simulink model "templateVFreplay"  (R2019b)
settings: Solver=ode23tb  StartTime=0  StopTime=dataSim(l).Time(end)  FixedStep=Ts
model workspace (MAT data in the model file):
  AC8B_test_sdosession : sldodialogs.data.SessionData (value not decoded)
  tp34291882_bceb_4da8_b486_81ba615ab517 = [0 0.0333333 0.0666667 0.1 0.1333334 0.1666667 0.2 0.2333333 0.2666666 0.2999999 0.3333332 0.3666665 ... (13500 elements, 2700x5)]
  tp5fd81924_c6b2_4820_a4c1_c746ac51258e : object (value not decoded)
  tp61e2f470_2812_498a_af75_e87b8b944307 = [0 0.0333333 0.0666667 0.1 0.1333334 0.1666667 0.2 0.2333333 0.2666666 0.2999999 0.3333332 0.3666665 ... (13500 elements, 2700x5)]
  tpfa3056f0_c430_45b3_969f_b76cef1498ad : object (value not decoded)
undefined symbols (not defined in the file): dataSim, dyn, Fnom, g, gcbh, genTpd0, genTppd0, genTppq0, genTpq0, genXd, genXl, genXpd, genXppd, genXppq, genXpq, genXq, govDisable, ifd, init, j, l, MBase, p, sps_rtmsupport, sys, Tb1, Tc1, Vnom, vt
libraries: powerlib x28, modelLibrary x22, simulink x15, powerlib_meascontrol x5, spsST2AModel x4, GenLib x2, ideal_source x1
(part 4 of 4)

== system templateVFreplay/VF Replay/AVR/ST4B/ST4B Excitation System (Continuous)/Fex ==
  note: In<=0.433        Case 3
      | 0.433<In<0.75 Case 2
      | 0.75<=In<=1.0 Case 1
      | In>1.0               default
  In : Inport
  0.433<In<0.75 : Subsystem  TreatAsAtomicUnit=on
  0.75<=In<=1.0 : Subsystem  TreatAsAtomicUnit=on
  In<=0.433 : Subsystem  TreatAsAtomicUnit=on
  In>1.0 : Subsystem  TreatAsAtomicUnit=on
  Merge : Merge  Inputs=4
  Relational Operator : RelationalOperator  Operator=<=  RndMeth=Nearest  InputSameDT=on
  Relational Operator1 : RelationalOperator  Operator=<  RndMeth=Nearest  InputSameDT=on
  Relational Operator2 : RelationalOperator  Operator=<=  RndMeth=Nearest  InputSameDT=on
  Sum : Sum  Inputs=+++  AccumDataTypeStr=double  OutDataTypeStr=double  SaturateOnIntegerOverflow=on  InputSameDT=on
  Switch Case : SwitchCase  CaseConditions={1 2 3}
  input : Constant  Value=0.433
  input1 : Constant  Value=0.75
  input2 : Constant  Value=1.0
  Fex : Outport  VectorParamsAs1DForOutWhenUnconnected=off
  wires:
  Merge/1 -> Fex/1
  In/1 -> Relational Operator2/1, 0.75<=In<=1.0/1(In), 0.433<In<0.75/1(In), In<=0.433/1(In), Relational Operator1/1, Relational Operator/1  "In"
  0.75<=In<=1.0/1(f(In)) -> Merge/1
  0.433<In<0.75/1(f(In)) -> Merge/2
  In>1.0/1(f(In)) -> Merge/4
  In<=0.433/1(f(In)) -> Merge/3
  input1/1 -> Relational Operator1/2
  input2/1 -> Relational Operator2/2
  Relational Operator1/1 -> Sum/2
  Relational Operator/1 -> Sum/1
  Relational Operator2/1 -> Sum/3
  Sum/1 -> Switch Case/1
  Switch Case/1 -> 0.75<=In<=1.0/Action
  Switch Case/2 -> 0.433<In<0.75/Action
  Switch Case/3 -> In<=0.433/Action
  Switch Case/4 -> In>1.0/Action
  input/1 -> Relational Operator/2

== system templateVFreplay/VF Replay/AVR/ST4B/ST4B Excitation System (Continuous)/Fex1 ==
  Ve : Inport
  Ifd : Inport  Port=2
  Fcn : Fcn  Expr=u+(u==0)*eps
  Gain : Gain  Gain=Kc  SaturateOnIntegerOverflow=on  OutDataTypeStr=Inherit: Same as input  ParamDataTypeStr=Inherit: Same as input
  Product : Product  Inputs=*/  SaturateOnIntegerOverflow=on  RndMeth=Zero  InputSameDT=on  OutDataTypeStr=Inherit: Same as first input
  IN : Outport  VectorParamsAs1DForOutWhenUnconnected=off
  wires:
  Product/1 -> Gain/1
  Ifd/1 -> Product/1
  Fcn/1 -> Product/2
  Ve/1 -> Fcn/1
  Gain/1 -> IN/1  "In"

== system templateVFreplay/VF Replay/AVR/ST4B/ST4B Excitation System (Continuous)/S1 ==
  In1 : Inport
  Gain2 : Gain  Gain=Kpr
  Gain3 : Gain  Gain=Kir
  Integrator (Anti-windup) : Subsystem
      mask Display: dpoly([1],[1 0],'s')
  Saturation1 : Saturate  UpperLimit=Vrmax  LowerLimit=Vrmin
  Sum2 : Sum  Inputs=|++
  Out1 : Outport  VectorParamsAs1DForOutWhenUnconnected=off
  wires:
  Gain3/1 -> Integrator (Anti-windup)/1(u)
  In1/1 -> Gain3/1, Gain2/1
  Integrator (Anti-windup)/1(Out2) -> Sum2/2
  Gain2/1 -> Sum2/1
  Sum2/1 -> Integrator (Anti-windup)/2(ctrlOutput1), Saturation1/1
  Saturation1/1 -> Out1/1

== system templateVFreplay/VF Replay/AVR/ST4B/ST4B Excitation System (Continuous)/Subsystem2 ==
  note: Kp*Vt
  Vt : Inport
  Vt_Ang : Inport  Port=2
  It : Inport  Port=3
  It_Ang : Inport  Port=4
  Complex to Magnitude : ComplexToMagnitudeAngle  Output=Magnitude
  Current Source Gain : Constant  Value=Ki
  Gain : Gain  Gain=j
  Leakage Reactance : Constant  Value=Xl
  Magnitude-Angle to Complex : MagnitudeAngleToComplex
  Magnitude-Angle to Complex1 : MagnitudeAngleToComplex
  Magnitude-Angle to Complex2 : MagnitudeAngleToComplex
  Potential Source Gain : Constant  Value=Kp
  Potential Source Phase Angle : Constant  Value=Angp
  Product1 : Product  SaturateOnIntegerOverflow=on  RndMeth=Zero  InputSameDT=on  OutDataTypeStr=Inherit: Same as first input
  Product2 : Product  SaturateOnIntegerOverflow=on  RndMeth=Zero  InputSameDT=on  OutDataTypeStr=Inherit: Same as first input
  Product3 : Product  SaturateOnIntegerOverflow=on  RndMeth=Zero  InputSameDT=on  OutDataTypeStr=Inherit: Same as first input
  Sum5 : Sum  Inputs=|++
  Sum6 : Sum  Inputs=++|
  Ve : Outport  VectorParamsAs1DForOutWhenUnconnected=off
  wires:
  Magnitude-Angle to Complex2/1 -> Product2/1
  Potential Source Phase Angle/1 -> Magnitude-Angle to Complex/2
  Magnitude-Angle to Complex1/1 -> Product1/2
  Potential Source Gain/1 -> Magnitude-Angle to Complex/1
  Product1/1 -> Sum5/1
  Product2/1 -> Sum5/2
  Sum5/1 -> Complex to Magnitude/1
  Vt/1 -> Magnitude-Angle to Complex1/1
  Complex to Magnitude/1 -> Ve/1  "Ve"
  Magnitude-Angle to Complex/1 -> Product3/1, Product1/1
  Leakage Reactance/1 -> Product3/2
  Product3/1 -> Sum6/2  "Kp*XL"
  Current Source Gain/1 -> Sum6/1
  Sum6/1 -> Gain/1  "Ki+Kp*XL"
  Gain/1 -> Product2/2
  It/1 -> Magnitude-Angle to Complex2/1
  Vt_Ang/1 -> Magnitude-Angle to Complex1/2
  It_Ang/1 -> Magnitude-Angle to Complex2/2

== system templateVFreplay/VF Replay/AVR/ST4B/ST4B Excitation System (Continuous)/Subsystem4 ==
  In1 : Inport
  Gain2 : Gain  Gain=Kpm
  Gain3 : Gain  Gain=Kim
  Integrator (Anti-windup) : Subsystem
      mask Display: dpoly([1],[1 0],'s')
  Saturation1 : Saturate  UpperLimit=Vmmax  LowerLimit=Vmmin
  Sum2 : Sum  Inputs=|++
  Out1 : Outport  VectorParamsAs1DForOutWhenUnconnected=off
  wires:
  Gain3/1 -> Integrator (Anti-windup)/1(u)
  Saturation1/1 -> Out1/1
  Gain2/1 -> Sum2/1
  Integrator (Anti-windup)/1(Out2) -> Sum2/2
  In1/1 -> Gain2/1, Gain3/1
  Sum2/1 -> Integrator (Anti-windup)/2(ctrlOutput1), Saturation1/1

== system templateVFreplay/VF Replay/AVR/ST4B/ST4B Excitation System (Continuous)/k//(tau.s+1)1 ==
  u : Inport
  1/(taus+1) : Subsystem  mask{tau=tau, vmax=vmax, vmin=vmin}
      mask prompts: tau "Time Constant"
      mask init:
      | h = gcbh;
      | 
      | qq = get(h,'MaskValues');
      | 
      | if eval(qq{1}) == 0
      |     
      |     set(h,'Commented','through');
      |     
      | else
      |     
      |     set(h,'Commented','off');
      |     
      | end
  k : Gain  Gain=k
  y : Outport  VectorParamsAs1DForOutWhenUnconnected=off
  wires:
  1/(taus+1)/1(y) -> y/1
  u/1 -> k/1
  k/1 -> 1/(taus+1)/1(u)

== system templateVFreplay/VF Replay/GENERATION/GENROU_TERMINAL/freqMeas/S0 ==
  u : Inport
  Gain : Gain  Gain=1/1e-2
  Gain1 : Gain  Gain=1e-2
  Integrator : Integrator
  Sum : Sum  Inputs=|+-
  y : Outport  InitialOutput=0  VectorParamsAs1DForOutWhenUnconnected=off
  wires:
  Gain1/1 -> y/1
  Integrator/1 -> Sum/2
  Gain/1 -> Integrator/1, Gain1/1
  Sum/1 -> Gain/1
  u/1 -> Sum/1

== system templateVFreplay/VF Replay/GENERATION/GENROU_TERMINAL/freqMeas/S1 ==
  u : Inport
  Gain2 : Gain  Gain=100
  Integrator1 : Integrator
  Sum : Sum  Inputs=|+-
  y : Outport  InitialOutput=0  VectorParamsAs1DForOutWhenUnconnected=off
  wires:
  u/1 -> Sum/1
  Sum/1 -> Gain2/1
  Integrator1/1 -> y/1, Sum/2
  Gain2/1 -> Integrator1/1

== system templateVFreplay/VF Replay/GENERATION/GENROU_TRANSFORMER/freqMeas/S0 ==
  u : Inport
  Gain : Gain  Gain=1/1e-2
  Gain1 : Gain  Gain=1e-2
  Integrator : Integrator
  Sum : Sum  Inputs=|+-
  y : Outport  InitialOutput=0  VectorParamsAs1DForOutWhenUnconnected=off
  wires:
  u/1 -> Sum/1
  Sum/1 -> Gain/1
  Gain/1 -> Gain1/1, Integrator/1
  Integrator/1 -> Sum/2
  Gain1/1 -> y/1

== system templateVFreplay/VF Replay/GENERATION/GENROU_TRANSFORMER/freqMeas/S1 ==
  u : Inport
  Gain2 : Gain  Gain=100
  Integrator1 : Integrator
  Sum : Sum  Inputs=|+-
  y : Outport  InitialOutput=0  VectorParamsAs1DForOutWhenUnconnected=off
  wires:
  Gain2/1 -> Integrator1/1
  Integrator1/1 -> Sum/2, y/1
  Sum/1 -> Gain2/1
  u/1 -> Sum/1

== system templateVFreplay/VF Replay/GENERATION/GENSAL_TRANSFORMER/freqMeas/S0 ==
  u : Inport
  Gain : Gain  Gain=1/1e-2
  Gain1 : Gain  Gain=1e-2
  Integrator : Integrator
  Sum : Sum  Inputs=|+-
  y : Outport  InitialOutput=0  VectorParamsAs1DForOutWhenUnconnected=off
  wires:
  Gain1/1 -> y/1
  Integrator/1 -> Sum/2
  Gain/1 -> Integrator/1, Gain1/1
  Sum/1 -> Gain/1
  u/1 -> Sum/1

== system templateVFreplay/VF Replay/GENERATION/GENSAL_TRANSFORMER/freqMeas/S1 ==
  u : Inport
  Gain2 : Gain  Gain=100
  Integrator1 : Integrator
  Sum : Sum  Inputs=|+-
  y : Outport  InitialOutput=0  VectorParamsAs1DForOutWhenUnconnected=off
  wires:
  u/1 -> Sum/1
  Sum/1 -> Gain2/1
  Integrator1/1 -> y/1, Sum/2
  Gain2/1 -> Integrator1/1

== system templateVFreplay/VF Replay/GENERATION/GENTPJ_TERMINAL/freqMeas/S0 ==
  u : Inport
  Gain : Gain  Gain=1/1e-2
  Gain1 : Gain  Gain=1e-2
  Integrator : Integrator
  Sum : Sum  Inputs=|+-
  y : Outport  InitialOutput=0  VectorParamsAs1DForOutWhenUnconnected=off
  wires:
  Gain1/1 -> y/1
  Integrator/1 -> Sum/2
  Gain/1 -> Integrator/1, Gain1/1
  Sum/1 -> Gain/1
  u/1 -> Sum/1

== system templateVFreplay/VF Replay/GENERATION/GENTPJ_TERMINAL/freqMeas/S1 ==
  u : Inport
  Gain2 : Gain  Gain=100
  Integrator1 : Integrator
  Sum : Sum  Inputs=|+-
  y : Outport  InitialOutput=0  VectorParamsAs1DForOutWhenUnconnected=off
  wires:
  u/1 -> Sum/1
  Sum/1 -> Gain2/1
  Integrator1/1 -> y/1, Sum/2
  Gain2/1 -> Integrator1/1

== system templateVFreplay/VF Replay/GENERATION/GENTPJ_TRANSFORMER/freqMeas/S0 ==
  u : Inport
  Gain : Gain  Gain=1/1e-2
  Gain1 : Gain  Gain=1e-2
  Integrator : Integrator
  Sum : Sum  Inputs=|+-
  y : Outport  InitialOutput=0  VectorParamsAs1DForOutWhenUnconnected=off
  wires:
  u/1 -> Sum/1
  Sum/1 -> Gain/1
  Gain/1 -> Gain1/1, Integrator/1
  Integrator/1 -> Sum/2
  Gain1/1 -> y/1

== system templateVFreplay/VF Replay/GENERATION/GENTPJ_TRANSFORMER/freqMeas/S1 ==
  u : Inport
  Gain2 : Gain  Gain=100
  Integrator1 : Integrator
  Sum : Sum  Inputs=|+-
  y : Outport  InitialOutput=0  VectorParamsAs1DForOutWhenUnconnected=off
  wires:
  Gain2/1 -> Integrator1/1
  Integrator1/1 -> Sum/2, y/1
  Sum/1 -> Gain2/1
  u/1 -> Sum/1

== system templateVFreplay/VF Replay/GOV/GGOV1/General Governor (Continuous) /Engine Power vs Speed ==
  u : Inport
  Droop3 : Gain  Gain=Dm
  Pmwset6 : Constant  Value=Dm
  Pmwset7 : Constant  Value=0
  Switch : Switch  Criteria=u2 > Threshold  ZeroCross=off
  y : Outport  VectorParamsAs1DForOutWhenUnconnected=off
  wires:
  u/1 -> Switch/1
  Droop3/1 -> y/1
  Switch/1 -> Droop3/1
  Pmwset7/1 -> Switch/3
  Pmwset6/1 -> Switch/2

== system templateVFreplay/VF Replay/GOV/GGOV1/General Governor (Continuous) /Fuel Flow Factor ==
  u : Inport
  Math Function : Math  Operator=pow  SaturateOnIntegerOverflow=on
  Pmwset6 : Constant  Value=Dm
  Pmwset7 : Constant  Value=0
  Pmwset8 : Constant  Value=Dm
  Switch : Switch  Criteria=u2 > Threshold  ZeroCross=off
  y : Outport  VectorParamsAs1DForOutWhenUnconnected=off
  wires:
  Pmwset7/1 -> Switch/1
  u/1 -> Switch/3
  Math Function/1 -> y/1
  Pmwset8/1 -> Math Function/2
  Switch/1 -> Math Function/1
  Pmwset6/1 -> Switch/2

== system templateVFreplay/VF Replay/GOV/GGOV1/General Governor (Continuous) /S0 ==
  In : Inport
  1/Tpelec : Gain  Gain=1/Tpelec
  Integrator : Integrator
  Sum : Sum  Inputs=|+-
  Out : Outport  InitialOutput=0  VectorParamsAs1DForOutWhenUnconnected=off
  wires:
  Sum/1 -> 1/Tpelec/1
  1/Tpelec/1 -> Integrator/1
  In/1 -> Sum/1
  Integrator/1 -> Sum/2, Out/1

== system templateVFreplay/VF Replay/GOV/GGOV1/General Governor (Continuous) /S1 ==
  u : Inport
  Droop1 : Gain  Gain=Kpgov
  S1_TF : Subsystem
      mask Display: disp('s K_{dgov} / (1 + s T_{dgov})','texmode','on');
  Sum4 : Sum  Inputs=++|
  y : Outport  InitialOutput=0  VectorParamsAs1DForOutWhenUnconnected=off
  wires:
  Sum4/1 -> y/1  "Pm0*Kpgov"
  S1_TF/1(y) -> Sum4/1  "0"
  Droop1/1 -> Sum4/2
  u/1 -> Droop1/1, S1_TF/1(u)

== system templateVFreplay/VF Replay/GOV/GGOV1/General Governor (Continuous) /S2 ==
  u : Inport
  Droop2 : Gain  Gain=Kigov/Kpgov
  Integrator : Integrator
  y : Outport  InitialOutput=0  VectorParamsAs1DForOutWhenUnconnected=off
  wires:
  Integrator/1 -> y/1
  Droop2/1 -> Integrator/1
  u/1 -> Droop2/1

== system templateVFreplay/VF Replay/GOV/GGOV1/General Governor (Continuous) /S3 ==
  u : Inport
  Droop2 : Gain  Gain=1/Tact
  Integrator : Integrator  InitialCondition=1
  Saturation3 : Saturate  Commented=through  UpperLimit=ropen  LowerLimit=rclose
      settings: AttributesFormatString=|
      | %<UpperLimit>
      | %<LowerLimit>
  y : Outport  InitialOutput=0  VectorParamsAs1DForOutWhenUnconnected=off
  wires:
  u/1 -> Droop2/1
  Droop2/1 -> Saturation3/1
  Saturation3/1 -> Integrator/1
  Integrator/1 -> y/1

== system templateVFreplay/VF Replay/GOV/GGOV1/General Governor (Continuous) /S4 ==
  u : Inport
  Gain : Gain  Gain=1/Tb
  Gain1 : Gain  Gain=Tc
  Integrator : Integrator  InitialCondition=1
  Sum : Sum  Inputs=|+-
  Sum1 : Sum  Inputs=++|
  y : Outport  InitialOutput=0  VectorParamsAs1DForOutWhenUnconnected=off
  wires:
  Sum1/1 -> y/1
  Gain/1 -> Integrator/1, Gain1/1
  Sum/1 -> Gain/1
  u/1 -> Sum/1  "Pm0"
  Integrator/1 -> Sum1/2, Sum/2
  Gain1/1 -> Sum1/1

== system templateVFreplay/VF Replay/GOV/GGOV1/General Governor (Continuous) /S5 ==
  u : Inport
  1/Tfload : Gain  Gain=1/Tfload
  Integrator : Integrator
  Sum : Sum  Inputs=|+-
  y : Outport  InitialOutput=0  VectorParamsAs1DForOutWhenUnconnected=off
  wires:
  Sum/1 -> 1/Tfload/1
  1/Tfload/1 -> Integrator/1
  u/1 -> Sum/1
  Integrator/1 -> Sum/2, y/1

== system templateVFreplay/VF Replay/GOV/GGOV1/General Governor (Continuous) /S6 ==
  u : Inport
  Droop2 : Gain  Gain=Kiload/Kpload
  Integrator : Integrator
  y : Outport  InitialOutput=0  VectorParamsAs1DForOutWhenUnconnected=off
  wires:
  u/1 -> Droop2/1
  Droop2/1 -> Integrator/1
  Integrator/1 -> y/1

== system templateVFreplay/VF Replay/GOV/GGOV1/General Governor (Continuous) /S7 ==
  u : Inport
  Gain1 : Gain  Gain=Kimw
  Integrator : Integrator  UpperSaturationLimit=1.1*r  LowerSaturationLimit=-1.1*r
      settings: AttributesFormatString=|
      | %<UpperSaturationLimit>
      | %<LowerSaturationLimit>
  y : Outport  InitialOutput=0  VectorParamsAs1DForOutWhenUnconnected=off
  wires:
  u/1 -> Gain1/1
  Gain1/1 -> Integrator/1
  Integrator/1 -> y/1

== system templateVFreplay/VF Replay/GOV/GGOV1/General Governor (Continuous) /S8 ==
  u : Inport
  Gain : Gain  Gain=1/Ta
  Integrator : Integrator
  Sum : Sum  Inputs=|+-
  y : Outport  InitialOutput=0  VectorParamsAs1DForOutWhenUnconnected=off
  wires:
  Gain/1 -> Integrator/1, y/1
  u/1 -> Sum/1
  Sum/1 -> Gain/1
  Integrator/1 -> Sum/2

== system templateVFreplay/VF Replay/GOV/GGOV1/General Governor (Continuous) /S9 ==
  u : Inport
  Gain : Gain  Gain=1/Tsb
  Gain1 : Gain  Gain=Tsa
  Integrator : Integrator
  Sum : Sum  Inputs=|+-
  Sum1 : Sum  Inputs=++|
  y : Outport  InitialOutput=0  VectorParamsAs1DForOutWhenUnconnected=off
  wires:
  Gain1/1 -> Sum1/1
  Integrator/1 -> Sum/2, Sum1/2
  u/1 -> Sum/1  "Pm0/Kturb+wfnl"
  Sum/1 -> Gain/1
  Gain/1 -> Integrator/1, Gain1/1
  Sum1/1 -> y/1

== system templateVFreplay/VF Replay/GOV/GGOV1/General Governor (Continuous) /Subsystem ==
  Clock : Clock
  Memory : Memory  InitialCondition=-0.2
  Sum13 : Sum  Inputs=|+-
  dT : Outport  VectorParamsAs1DForOutWhenUnconnected=off
  wires:
  Sum13/1 -> dT/1
  Clock/1 -> Sum13/1, Memory/1
  Memory/1 -> Sum13/2

== system templateVFreplay/VF Replay/GOV/GGOV1/General Governor (Continuous) /Subsystem1 ==
  fsrt : Inport
  fsra : Inport  Port=2
  fsrn : Inport  Port=3
  Constant : Constant  Value=init*100
  Low Value Select : MinMax  Inputs=3  ZeroCross=off
  Sum : Sum  Inputs=|+-
  Sum1 : Sum  Inputs=|++
  Unit Delay : UnitDelay  SampleTime=-1  HasFrameUpgradeWarning=on
  Out1 : Outport  VectorParamsAs1DForOutWhenUnconnected=off
  wires:
  fsra/1 -> Low Value Select/2
  fsrt/1 -> Low Value Select/1
  Unit Delay/1 -> Out1/1
  fsrn/1 -> Sum/1
  Sum/1 -> Low Value Select/3
  Low Value Select/1 -> Sum1/1
  Sum1/1 -> Unit Delay/1
  Constant/1 -> Sum1/2, Sum/2

== system templateVFreplay/VF Replay/GOV/IEEEG3/Hydro Turbine//Governor (Continuous)/S0 ==
  u : Inport
  1/Tp : Gain  Gain=1/Tp
  Integrator : Integrator
  Sum : Sum  Inputs=|+-
  y : Outport  VectorParamsAs1DForOutWhenUnconnected=off
  wires:
  Integrator/1 -> y/1, Sum/2
  u/1 -> Sum/1
  1/Tp/1 -> Integrator/1
  Sum/1 -> 1/Tp/1

== system templateVFreplay/VF Replay/GOV/IEEEG3/Hydro Turbine//Governor (Continuous)/S2 ==
  u : Inport
  Gain : Gain  Gain=1/Tr
  Gain1 : Gain  Gain=Tr
  Gain2 : Gain  Gain=Rtemp
  Integrator : Integrator
  Sum : Sum  Inputs=|+-
  y : Outport  InitialOutput=0  VectorParamsAs1DForOutWhenUnconnected=off
  wires:
  Gain1/1 -> y/1
  Integrator/1 -> Sum/2
  Gain/1 -> Gain1/1, Integrator/1
  Sum/1 -> Gain/1
  u/1 -> Gain2/1
  Gain2/1 -> Sum/1

== system templateVFreplay/VF Replay/GOV/IEEEG3/Hydro Turbine//Governor (Continuous)/S3 ==
  u : Inport
  Gain : Gain  Gain=1/(Bturb*Tw)
  Gain1 : Gain  Gain=Aturb*Tw
  Gain2 : Gain  Gain=Kturb
  Integrator : Integrator  InitialCondition=1
  Sum : Sum  Inputs=|+-
  Sum1 : Sum  Inputs=++|
  y : Outport  InitialOutput=0  VectorParamsAs1DForOutWhenUnconnected=off
  wires:
  u/1 -> Gain2/1
  Sum1/1 -> y/1
  Gain/1 -> Gain1/1, Integrator/1
  Sum/1 -> Gain/1
  Gain2/1 -> Sum/1
  Integrator/1 -> Sum1/2, Sum/2
  Gain1/1 -> Sum1/1

== system templateVFreplay/VF Replay/PSS/PSS1A/Power System Stabilize 1A (Continuous)/(ta.s+1)//(tb.s+1)1 ==
  note: disable integrator and pass through signal if tb is zero
  u : Inport
  Constant : Constant  Value=tb
  Gain : Gain  Gain=1/(tb+eps)
  Gain1 : Gain  Gain=ta
  Integrator : Integrator
  Sum : Sum  Inputs=|+-
  Sum1 : Sum  Inputs=++|
  Switch : Switch  Criteria=u2 > Threshold
  Switch1 : Switch  Criteria=u2 > Threshold
  y : Outport  VectorParamsAs1DForOutWhenUnconnected=off
  wires:
  Switch1/1 -> y/1
  Sum1/1 -> Switch1/1
  Switch/1 -> Integrator/1
  Constant/1 -> Switch/2, Switch/3, Switch1/2
  u/1 -> Sum/1, Switch1/3
  Integrator/1 -> Sum/2, Sum1/2
  Gain1/1 -> Sum1/1
  Gain/1 -> Gain1/1, Switch/1
  Sum/1 -> Gain/1

== system templateVFreplay/VF Replay/PSS/PSS1A/Power System Stabilize 1A (Continuous)/S3_1 ==
  u : Inport
  1/A1 : Gain  Gain=1/A1
  Gain3 : Gain  Commented=on  Gain=A1/A2
  Gain4 : Gain  Commented=on  Gain=1/A2
  Gain5 : Gain  Commented=on  Gain=1/A2
  Integrator : Integrator
  Integrator2 : Integrator  Commented=on
  Integrator3 : Integrator  Commented=on
  Sum : Sum  Inputs=|+-
  Sum2 : Sum  Commented=on  Inputs=|+-
  Sum3 : Sum  Commented=on  Inputs=|++
  y : Outport  InitialOutput=0  VectorParamsAs1DForOutWhenUnconnected=off
  wires:
  Integrator/1 -> Sum/2, y/1
  u/1 -> Sum/1
  1/A1/1 -> Integrator/1
  Sum/1 -> 1/A1/1
  Gain4/1 -> Sum3/1
  Gain3/1 -> Sum3/2
  Sum3/1 -> Sum2/2  "Vs0/A2"
  Gain5/1 -> Sum2/1
  Sum2/1 -> Integrator2/1
  Integrator2/1 -> Gain3/1, Integrator3/1
  Integrator3/1 -> Gain4/1
  ? -> Gain5/1

== system templateVFreplay/VF Replay/PSS/PSS2A/Power System Stabilizer 2A (Continuous) /T9 ~= 0 ==
  u : Inport
  Filter1 : Subsystem
      mask Display: disp('(1 + s T_8) / (1 + s T_9)^m','texmode','on');
  y : Outport  VectorParamsAs1DForOutWhenUnconnected=off
  wires:
  u/1 -> Filter1/1(In1)
  Filter1/1(Out1) -> y/1

== system templateVFreplay/VF Replay/PSS/PSS2B/Power System Stabilizer 2B (Continuous) /T9 ~= 0 ==
  u : Inport
  Filter1 : Subsystem
      mask Display: disp('(1 + s T_8) / (1 + s T_9)^m','texmode','on');
  y : Outport  VectorParamsAs1DForOutWhenUnconnected=off
  wires:
  u/1 -> Filter1/1(In1)
  Filter1/1(Out1) -> y/1

== system templateVFreplay/VF Replay/AVR/REXS/Rotating Excitation System (Continuous) /S2 + S8/S2 ==
  In : Inport
  Tb1 = 0 : Subsystem  VariantControl=Tb1Zero
  Tb1 ~= 0 : Subsystem  VariantControl=Tb1NotZero
  Out : Outport  VectorParamsAs1DForOutWhenUnconnected=off

== system templateVFreplay/VF Replay/AVR/REXS/Rotating Excitation System (Continuous) /S2 + S8/S8 ==
  In : Inport
  Tb2 = 0 : Subsystem  VariantControl=Tb2Zero
  Tb2 ~= 0 : Subsystem  VariantControl=Tb2NotZero
  Out : Outport  VectorParamsAs1DForOutWhenUnconnected=off

== system templateVFreplay/VF Replay/AVR/ST1A/ST1A Excitation System/Model/(ta.s+1)//(tb.s+1)1 ==
  note: disable integrator and pass through signal if tb is zero
  u : Inport
  Constant : Constant  Value=tb
  Gain : Gain  Gain=1/(tb+eps)
  Gain1 : Gain  Gain=ta
  Integrator : Integrator
  Sum : Sum  Inputs=|+-
  Sum1 : Sum  Inputs=++|
  Switch : Switch  Criteria=u2 > Threshold
  Switch1 : Switch  Criteria=u2 > Threshold
  y : Outport  VectorParamsAs1DForOutWhenUnconnected=off
  wires:
  Switch1/1 -> y/1
  Sum1/1 -> Switch1/1
  Switch/1 -> Integrator/1
  Constant/1 -> Switch/2, Switch/3, Switch1/2
  u/1 -> Sum/1, Switch1/3
  Integrator/1 -> Sum/2, Sum1/2
  Gain1/1 -> Sum1/1
  Gain/1 -> Gain1/1, Switch/1
  Sum/1 -> Gain/1

== system templateVFreplay/VF Replay/AVR/ST1A/ST1A Excitation System/Model/Subsystem ==
  note: Vt.VRmin
  Efd : Inport
  Vt : Inport  Port=2
  Ifd : Inport  Port=3
  Gain2 : Gain  Gain=p.kc  SaturateOnIntegerOverflow=on  OutDataTypeStr=Inherit: Same as input  ParamDataTypeStr=Inherit: Same as input
  Gain5 : Gain  Gain=p.vrmax  SaturateOnIntegerOverflow=on  OutDataTypeStr=Inherit: Same as input  ParamDataTypeStr=Inherit: Same as input
  Gain6 : Gain  Gain=p.vrmin  SaturateOnIntegerOverflow=on  OutDataTypeStr=Inherit: Same as input  ParamDataTypeStr=Inherit: Same as input
  Saturation Dynamic : simulink/Discontinuities/Saturation Dynamic  OutMin=[]  OutMax=[]  OutDataTypeStr=Inherit: Same as second input  OutDataType=fixdt(1, 16)  OutScaling=2^-10  DoSatur=off
  Sum5 : Sum  Inputs=+-  SaturateOnIntegerOverflow=on  InputSameDT=on  OutDataTypeStr=Inherit: Same as first input
  Efd1 : Outport  VectorParamsAs1DForOutWhenUnconnected=off
  wires:
  Gain2/1 -> Sum5/2
  Ifd/1 -> Gain2/1  "Field current Ifd (pu)"
  Efd/1 -> Saturation Dynamic/2  "Field voltage Efd (pu)"
  Gain5/1 -> Sum5/1
  Vt/1 -> Gain6/1, Gain5/1  "Terminal voltage Vt (pu)"
  Saturation Dynamic/1 -> Efd1/1
  Sum5/1 -> Saturation Dynamic/1
  Gain6/1 -> Saturation Dynamic/3

== system templateVFreplay/VF Replay/AVR/ST1A/ST1A Excitation System/Model/const ==
  Constant : Constant  Value=0
  Integrator : Integrator
  y : Outport  VectorParamsAs1DForOutWhenUnconnected=off
  wires:
  Constant/1 -> Integrator/1
  Integrator/1 -> y/1

== system templateVFreplay/VF Replay/AVR/ST1A/ST1A Excitation System/Model/k.s//(tau.s+1) ==
  note: disable integrator and pass through signal if tau is zero
  u : Inport
  Constant : Constant  Value=tau
  Constant1 : Constant  Value=0
  Gain : Gain  Gain=1/(tau+eps)
  Gain1 : Gain  Gain=k
  Integrator : Integrator
  Sum : Sum  Inputs=|+-
  Switch : Switch  Criteria=u2 > Threshold
  Switch1 : Switch  Criteria=u2 > Threshold
  y : Outport  VectorParamsAs1DForOutWhenUnconnected=off
  wires:
  Gain1/1 -> Switch1/1
  Switch1/1 -> y/1
  Switch/1 -> Gain1/1, Integrator/1
  Gain/1 -> Switch/1
  Constant/1 -> Switch/2, Switch/3, Switch1/2
  Sum/1 -> Gain/1
  u/1 -> Sum/1
  Integrator/1 -> Sum/2
  Constant1/1 -> Switch1/3

== system templateVFreplay/VF Replay/AVR/ST1A/ST1A Excitation System/Model/k//(tau.s+1)1 ==
  u : Inport
  1/(taus+1) : Subsystem  mask{tau=tau, vmax=vmax, vmin=vmin}
      mask prompts: tau "Time Constant"
  k : Gain  Gain=k
  y : Outport  VectorParamsAs1DForOutWhenUnconnected=off
  wires:
  k/1 -> 1/(taus+1)/1(u)
  u/1 -> k/1
  1/(taus+1)/1(y) -> y/1

== system templateVFreplay/VF Replay/AVR/ST4B/ST4B Excitation System (Continuous)/Fex/0.433<In<0.75 ==
  In : Inport
  Action Port : ActionPort  InitializeStates=reset  ActionPortLabel=case [ 2 ]:
  Math Function : Math  Operator=square  SaturateOnIntegerOverflow=on
  Math Function1 : Math  Operator=sqrt  SaturateOnIntegerOverflow=on
  Sum : Sum  Inputs=+-|  SaturateOnIntegerOverflow=on  InputSameDT=on  OutDataTypeStr=Inherit: Same as first input
  input2 : Constant  Value=0.75
  f(In) : Outport  VectorParamsAs1DForOutWhenUnconnected=off
  wires:
  Math Function1/1 -> f(In)/1
  In/1 -> Math Function/1
  Math Function/1 -> Sum/2
  input2/1 -> Sum/1
  Sum/1 -> Math Function1/1

== system templateVFreplay/VF Replay/AVR/ST4B/ST4B Excitation System (Continuous)/Fex/0.75<=In<=1.0 ==
  In : Inport
  Action Port : ActionPort  InitializeStates=reset  ActionPortLabel=case [ 1 ]:
  Gain : Gain  Gain=1.732  SaturateOnIntegerOverflow=on  OutDataTypeStr=Inherit: Same as input  ParamDataTypeStr=Inherit: Same as input
  Sum : Sum  Inputs=+-|  SaturateOnIntegerOverflow=on  InputSameDT=on  OutDataTypeStr=Inherit: Same as first input
  input2 : Constant  Value=1.0
  f(In) : Outport  VectorParamsAs1DForOutWhenUnconnected=off
  wires:
  Gain/1 -> f(In)/1
  Sum/1 -> Gain/1
  input2/1 -> Sum/1
  In/1 -> Sum/2

== system templateVFreplay/VF Replay/AVR/ST4B/ST4B Excitation System (Continuous)/Fex/In<=0.433 ==
  In : Inport
  Action Port : ActionPort  InitializeStates=reset  ActionPortLabel=case [ 3 ]:
  Gain : Gain  Gain=0.577  SaturateOnIntegerOverflow=on  OutDataTypeStr=Inherit: Same as input  ParamDataTypeStr=Inherit: Same as input
  Sum : Sum  Inputs=+-|  SaturateOnIntegerOverflow=on  InputSameDT=on  OutDataTypeStr=Inherit: Same as first input
  input2 : Constant  Value=1.0
  f(In) : Outport  VectorParamsAs1DForOutWhenUnconnected=off
  wires:
  Sum/1 -> f(In)/1
  input2/1 -> Sum/1
  Gain/1 -> Sum/2
  In/1 -> Gain/1

== system templateVFreplay/VF Replay/AVR/ST4B/ST4B Excitation System (Continuous)/Fex/In>1.0 ==
  Action Port : ActionPort  InitializeStates=reset  ActionPortLabel=default:
  input2 : Constant  Value=0
  f(In) : Outport  InitialOutput=0  VectorParamsAs1DForOutWhenUnconnected=off
  wires:
  input2/1 -> f(In)/1

== system templateVFreplay/VF Replay/AVR/ST4B/ST4B Excitation System (Continuous)/S1/Integrator (Anti-windup) ==
  u : Inport
  ctrlOutput1 : Inport  Port=2
  Compare To Constant : simulink/Logic and Bit Operations/Compare To Constant  relop=>=  const=Vrmax  OutDataTypeStr=boolean
  Compare To Constant1 : simulink/Logic and Bit Operations/Compare To Constant  relop=<=  const=Vrmin  OutDataTypeStr=boolean
  Constant : Constant  Value=0
  Integrator : Integrator
  Logical Operator : Logic  Operator=OR  AllPortsSameDT=off  OutDataTypeStr=boolean
  Switch : Switch  Criteria=u2 > Threshold
  Out2 : Outport  VectorParamsAs1DForOutWhenUnconnected=off
  wires:
  Constant/1 -> Switch/1
  u/1 -> Switch/3
  Switch/1 -> Integrator/1
  Integrator/1 -> Out2/1
  Logical Operator/1 -> Switch/2
  ctrlOutput1/1 -> Compare To Constant1/1, Compare To Constant/1
  Compare To Constant/1 -> Logical Operator/1
  Compare To Constant1/1 -> Logical Operator/2

== system templateVFreplay/VF Replay/AVR/ST4B/ST4B Excitation System (Continuous)/Subsystem4/Integrator (Anti-windup) ==
  u : Inport
  ctrlOutput1 : Inport  Port=2
  Compare To Constant : simulink/Logic and Bit Operations/Compare To Constant  relop=>=  const=Vmmax  OutDataTypeStr=boolean
  Compare To Constant1 : simulink/Logic and Bit Operations/Compare To Constant  relop=<=  const=Vmmin  OutDataTypeStr=boolean
  Constant : Constant  Value=0
  Integrator : Integrator  InitialCondition=1
  Logical Operator : Logic  Operator=OR  AllPortsSameDT=off  OutDataTypeStr=boolean
  Switch : Switch  Criteria=u2 > Threshold
  Out2 : Outport  VectorParamsAs1DForOutWhenUnconnected=off
  wires:
  Integrator/1 -> Out2/1
  Switch/1 -> Integrator/1
  u/1 -> Switch/3
  Constant/1 -> Switch/1
  Logical Operator/1 -> Switch/2
  ctrlOutput1/1 -> Compare To Constant1/1, Compare To Constant/1
  Compare To Constant/1 -> Logical Operator/1
  Compare To Constant1/1 -> Logical Operator/2

== system templateVFreplay/VF Replay/AVR/ST4B/ST4B Excitation System (Continuous)/k//(tau.s+1)1/1//(taus+1) ==
  note: disable integrator and pass through signal if tau is zero
  u : Inport
  Constant : Constant  Value=tau
  Gain1 : Gain  Gain=1/(tau+eps)  SaturateOnIntegerOverflow=on  OutDataTypeStr=Inherit: Same as input  ParamDataTypeStr=Inherit: Same as input
  Integrator : Integrator  LimitOutput=on  UpperSaturationLimit=vmax  LowerSaturationLimit=vmin
  Sum : Sum  Inputs=|+-  SaturateOnIntegerOverflow=on  InputSameDT=on  OutDataTypeStr=Inherit: Same as first input
  Switch : Switch  Criteria=u2 > Threshold
  Switch1 : Switch  Criteria=u2 > Threshold
  y : Outport  VectorParamsAs1DForOutWhenUnconnected=off
  wires:
  Switch1/1 -> y/1
  Switch/1 -> Integrator/1
  Gain1/1 -> Switch/1
  Constant/1 -> Switch/2, Switch1/2, Switch/3
  Integrator/1 -> Switch1/1, Sum/2
  Sum/1 -> Gain1/1
  u/1 -> Sum/1, Switch1/3

== system templateVFreplay/VF Replay/GOV/GGOV1/General Governor (Continuous) /S1/S1_TF ==
  u : Inport
  Gain : Gain  Gain=1/Tdgov
  Gain1 : Gain  Gain=Kdgov
  Integrator : Integrator  InitialCondition=-Pmwset*r
  Sum : Sum  Inputs=|+-
  y : Outport  VectorParamsAs1DForOutWhenUnconnected=off
  wires:
  Gain1/1 -> y/1
  u/1 -> Sum/1
  Sum/1 -> Gain/1
  Integrator/1 -> Sum/2
  Gain/1 -> Integrator/1, Gain1/1

== system templateVFreplay/VF Replay/PSS/PSS2A/Power System Stabilizer 2A (Continuous) /T9 ~= 0/Filter1 ==
  In1 : Inport
  TF1 : Subsystem
      mask Display: disp('(1 + s T_8) / (1 + s T_9)','texmode','on');
  TF2 : Subsystem
      mask Display: disp('1 / (1 + s T_9)','texmode','on');
  TF3 : Subsystem
      mask Display: disp('1 / (1 + s T_9)','texmode','on');
  TF4 : Subsystem
      mask Display: disp('1 / (1 + s T_9)','texmode','on');
  TF5 : Subsystem
      mask Display: disp('1 / (1 + s T_9)','texmode','on');
  Out1 : Outport  VectorParamsAs1DForOutWhenUnconnected=off
  wires:
  In1/1 -> TF5/1(In1)
  TF5/1(Out1) -> TF4/1(In1)
  TF4/1(Out1) -> TF3/1(In1)
  TF3/1(Out1) -> TF2/1(In1)
  TF2/1(Out1) -> TF1/1(In1)
  TF1/1(Out1) -> Out1/1

== system templateVFreplay/VF Replay/PSS/PSS2B/Power System Stabilizer 2B (Continuous) /T9 ~= 0/Filter1 ==
  In1 : Inport
  TF1 : Subsystem
      mask Display: disp('(1 + s T_8) / (1 + s T_9)','texmode','on');
  TF2 : Subsystem
      mask Display: disp('1 / (1 + s T_9)','texmode','on');
  TF3 : Subsystem
      mask Display: disp('1 / (1 + s T_9)','texmode','on');
  TF4 : Subsystem
      mask Display: disp('1 / (1 + s T_9)','texmode','on');
  TF5 : Subsystem
      mask Display: disp('1 / (1 + s T_9)','texmode','on');
  Out1 : Outport  VectorParamsAs1DForOutWhenUnconnected=off
  wires:
  In1/1 -> TF5/1(In1)
  TF5/1(Out1) -> TF4/1(In1)
  TF4/1(Out1) -> TF3/1(In1)
  TF3/1(Out1) -> TF2/1(In1)
  TF2/1(Out1) -> TF1/1(In1)
  TF1/1(Out1) -> Out1/1

== system templateVFreplay/VF Replay/AVR/REXS/Rotating Excitation System (Continuous) /S2 + S8/S2/Tb1 = 0 ==
  In : Inport
  Out : Outport  VectorParamsAs1DForOutWhenUnconnected=off
  wires:
  In/1 -> Out/1

== system templateVFreplay/VF Replay/AVR/REXS/Rotating Excitation System (Continuous) /S2 + S8/S2/Tb1 ~= 0 ==
  In : Inport
  Gain : Gain  Gain=1/Tb1
  Gain1 : Gain  Gain=Tc1
  Integrator : Integrator
  Sum : Sum  Inputs=|+-
  Sum1 : Sum  Inputs=++|
  Out : Outport  InitialOutput=0  VectorParamsAs1DForOutWhenUnconnected=off
  wires:
  Gain1/1 -> Sum1/1
  Integrator/1 -> Sum/2, Sum1/2
  Sum/1 -> Gain/1
  Gain/1 -> Integrator/1, Gain1/1
  Sum1/1 -> Out/1
  In/1 -> Sum/1

== system templateVFreplay/VF Replay/AVR/REXS/Rotating Excitation System (Continuous) /S2 + S8/S8/Tb2 = 0 ==
  In : Inport
  Out : Outport  VectorParamsAs1DForOutWhenUnconnected=off
  wires:
  In/1 -> Out/1

== system templateVFreplay/VF Replay/AVR/REXS/Rotating Excitation System (Continuous) /S2 + S8/S8/Tb2 ~= 0 ==
  In : Inport
  Gain : Gain  Gain=1/Tb2
  Gain1 : Gain  Gain=Tc2
  Integrator : Integrator
  Sum : Sum  Inputs=|+-
  Sum1 : Sum  Inputs=++|
  Out : Outport  InitialOutput=0  VectorParamsAs1DForOutWhenUnconnected=off
  wires:
  Gain1/1 -> Sum1/1
  Integrator/1 -> Sum/2, Sum1/2
  Sum/1 -> Gain/1
  Gain/1 -> Integrator/1, Gain1/1
  Sum1/1 -> Out/1
  In/1 -> Sum/1

== system templateVFreplay/VF Replay/AVR/ST1A/ST1A Excitation System/Model/k//(tau.s+1)1/1//(taus+1) ==
  note: disable integrator and pass through signal if tau is zero
  u : Inport
  Constant : Constant  Value=tau
  Gain1 : Gain  Gain=1/(tau+eps)  SaturateOnIntegerOverflow=on  OutDataTypeStr=Inherit: Same as input  ParamDataTypeStr=Inherit: Same as input
  Integrator : Integrator  LimitOutput=on  UpperSaturationLimit=vmax  LowerSaturationLimit=vmin
  Sum : Sum  Inputs=|+-  SaturateOnIntegerOverflow=on  InputSameDT=on  OutDataTypeStr=Inherit: Same as first input
  Switch : Switch  Criteria=u2 > Threshold
  Switch1 : Switch  Criteria=u2 > Threshold
  y : Outport  VectorParamsAs1DForOutWhenUnconnected=off
  wires:
  u/1 -> Switch1/3, Sum/1
  Sum/1 -> Gain1/1
  Integrator/1 -> Sum/2, Switch1/1
  Constant/1 -> Switch/3, Switch1/2, Switch/2
  Gain1/1 -> Switch/1
  Switch/1 -> Integrator/1
  Switch1/1 -> y/1

== system templateVFreplay/VF Replay/PSS/PSS2A/Power System Stabilizer 2A (Continuous) /T9 ~= 0/Filter1/TF1 ==
  In1 : Inport
  Add : Sum
  Integrator : Integrator
  Sum : Sum  Inputs=|+-
  T8 : Gain  Gain=T8
  T9 : Gain  Gain=1/T9
  Out1 : Outport  VectorParamsAs1DForOutWhenUnconnected=off
  wires:
  Add/1 -> Out1/1
  T8/1 -> Add/1
  Integrator/1 -> Add/2, Sum/2
  T9/1 -> T8/1, Integrator/1
  Sum/1 -> T9/1
  In1/1 -> Sum/1

== system templateVFreplay/VF Replay/PSS/PSS2A/Power System Stabilizer 2A (Continuous) /T9 ~= 0/Filter1/TF2 ==
  In1 : Inport
  Integrator : Integrator
  Sum : Sum  Inputs=|+-
  T9 : Gain  Gain=1/T9
  Out1 : Outport  VectorParamsAs1DForOutWhenUnconnected=off
  wires:
  Integrator/1 -> Out1/1, Sum/2
  T9/1 -> Integrator/1
  Sum/1 -> T9/1
  In1/1 -> Sum/1

== system templateVFreplay/VF Replay/PSS/PSS2A/Power System Stabilizer 2A (Continuous) /T9 ~= 0/Filter1/TF3 ==
  In1 : Inport
  Integrator : Integrator
  Sum : Sum  Inputs=|+-
  T9 : Gain  Gain=1/T9
  Out1 : Outport  VectorParamsAs1DForOutWhenUnconnected=off
  wires:
  Integrator/1 -> Out1/1, Sum/2
  T9/1 -> Integrator/1
  Sum/1 -> T9/1
  In1/1 -> Sum/1

== system templateVFreplay/VF Replay/PSS/PSS2A/Power System Stabilizer 2A (Continuous) /T9 ~= 0/Filter1/TF4 ==
  In1 : Inport
  Integrator : Integrator
  Sum : Sum  Inputs=|+-
  T9 : Gain  Gain=1/T9
  Out1 : Outport  VectorParamsAs1DForOutWhenUnconnected=off
  wires:
  Integrator/1 -> Out1/1, Sum/2
  T9/1 -> Integrator/1
  Sum/1 -> T9/1
  In1/1 -> Sum/1

== system templateVFreplay/VF Replay/PSS/PSS2A/Power System Stabilizer 2A (Continuous) /T9 ~= 0/Filter1/TF5 ==
  In1 : Inport
  Integrator : Integrator
  Sum : Sum  Inputs=|+-
  T9 : Gain  Gain=1/T9
  Out1 : Outport  VectorParamsAs1DForOutWhenUnconnected=off
  wires:
  Integrator/1 -> Out1/1, Sum/2
  T9/1 -> Integrator/1
  Sum/1 -> T9/1
  In1/1 -> Sum/1

== system templateVFreplay/VF Replay/PSS/PSS2B/Power System Stabilizer 2B (Continuous) /T9 ~= 0/Filter1/TF1 ==
  In1 : Inport
  Add : Sum
  Integrator : Integrator
  Sum : Sum  Inputs=|+-
  T8 : Gain  Gain=T8
  T9 : Gain  Gain=1/T9
  Out1 : Outport  VectorParamsAs1DForOutWhenUnconnected=off
  wires:
  Add/1 -> Out1/1
  T8/1 -> Add/1
  Integrator/1 -> Add/2, Sum/2
  T9/1 -> T8/1, Integrator/1
  Sum/1 -> T9/1
  In1/1 -> Sum/1

== system templateVFreplay/VF Replay/PSS/PSS2B/Power System Stabilizer 2B (Continuous) /T9 ~= 0/Filter1/TF2 ==
  In1 : Inport
  Integrator : Integrator
  Sum : Sum  Inputs=|+-
  T9 : Gain  Gain=1/T9
  Out1 : Outport  VectorParamsAs1DForOutWhenUnconnected=off
  wires:
  Integrator/1 -> Out1/1, Sum/2
  T9/1 -> Integrator/1
  Sum/1 -> T9/1
  In1/1 -> Sum/1

== system templateVFreplay/VF Replay/PSS/PSS2B/Power System Stabilizer 2B (Continuous) /T9 ~= 0/Filter1/TF3 ==
  In1 : Inport
  Integrator : Integrator
  Sum : Sum  Inputs=|+-
  T9 : Gain  Gain=1/T9
  Out1 : Outport  VectorParamsAs1DForOutWhenUnconnected=off
  wires:
  Integrator/1 -> Out1/1, Sum/2
  T9/1 -> Integrator/1
  Sum/1 -> T9/1
  In1/1 -> Sum/1

== system templateVFreplay/VF Replay/PSS/PSS2B/Power System Stabilizer 2B (Continuous) /T9 ~= 0/Filter1/TF4 ==
  In1 : Inport
  Integrator : Integrator
  Sum : Sum  Inputs=|+-
  T9 : Gain  Gain=1/T9
  Out1 : Outport  VectorParamsAs1DForOutWhenUnconnected=off
  wires:
  Integrator/1 -> Out1/1, Sum/2
  T9/1 -> Integrator/1
  Sum/1 -> T9/1
  In1/1 -> Sum/1

== system templateVFreplay/VF Replay/PSS/PSS2B/Power System Stabilizer 2B (Continuous) /T9 ~= 0/Filter1/TF5 ==
  In1 : Inport
  Integrator : Integrator
  Sum : Sum  Inputs=|+-
  T9 : Gain  Gain=1/T9
  Out1 : Outport  VectorParamsAs1DForOutWhenUnconnected=off
  wires:
  Integrator/1 -> Out1/1, Sum/2
  T9/1 -> Integrator/1
  Sum/1 -> T9/1
  In1/1 -> Sum/1
